simulink model "Trajectory_Tracking_comparison_v22b"  (R2022b)
settings: Solver=VariableStepAuto  StartTime=0.0  StopTime=100  RelTol=1e-3
undefined symbols (not defined in the file): A, A_uns, B, B_uns, den_phi, den_theta, K_lq_track, K_lq_track_uns, K_lq_uns, K_pp, K_pp_uns, Kd_theta, Ki_phi, Ki_theta, Kp_phi, Kp_theta, num_phi, num_theta, Va_bar, x1_bar, x1_bar_uns, x3_bar, x3_bar_uns
libraries: simulink_extras x13, slpidlib x2, simulink x1
settings Model: Creator=Mark  LastModifiedBy=Mark
settings OptimizationCC: ReuseModelBlockBuffer=on

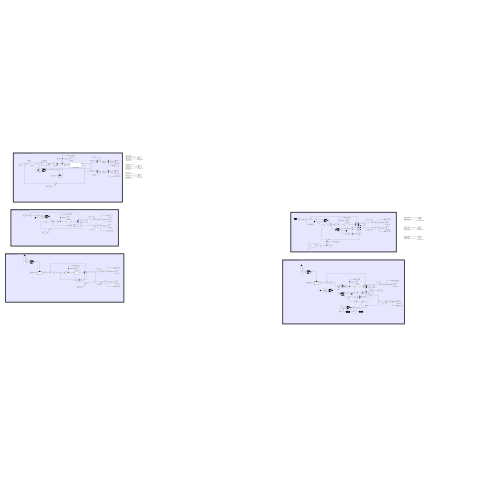
[thumbnail: Simulink's stored preview of the top-level diagram]
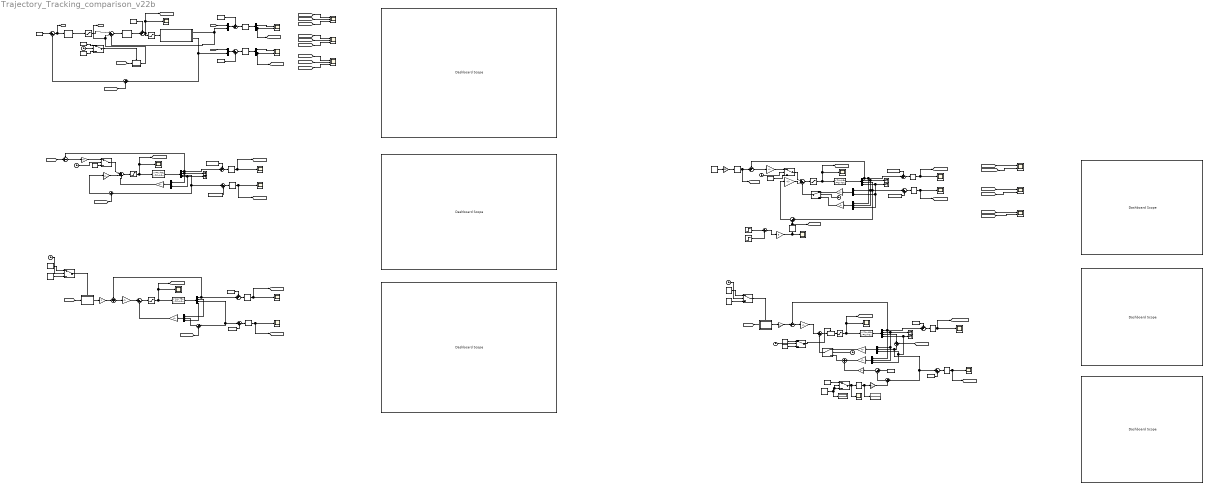
== system Trajectory_Tracking_comparison_v22b ==
  note: LQR + Trajectory Tracking at 0°
  note: LQR + Tracking Control for theta at 180°
  note: 2-DOF PID + Trajectory Tracking Control at 0°
  note: Pole Placement + Trajectory Tracking at 180°
  note: Pole Placement + Trajectory Tracking at 0°
  Clock{,1..7} (8 alike) : Clock
  Constant : Constant  Value=x3_bar_uns
  Constant1 : Constant  Value=x1_bar_uns
  Constant{2,6,10..11} (4 alike) : Constant
  Constant{3,7,12..13,19,22} (6 alike) : Constant  Value=0
  Constant14 : Constant  Value=Va_bar
  Constant15 : Constant  Value=x3_bar
  Constant16 : Constant  Value=x1_bar
  Constant17 : Constant  Value=x3_bar_uns
  Constant18 : Constant  Value=x1_bar_uns
  Constant20 : Constant  Value=x3_bar
  Constant21 : Constant  Value=x1_bar
  Constant4 : Constant  Value=pi
  Constant5 : Constant  Value=180
  Constant8 : Constant  Value=x3_bar
  Constant9 : Constant  Value=x1_bar
  Dashboard Scope{,1..5} (6 alike) : DashboardScope
  Degrees to Radians2 : simulink_extras/Transformations/Degrees to Radians
  Degrees to Radians7 : simulink_extras/Transformations/Degrees to Radians
  Degrees to Radians8 : simulink_extras/Transformations/Degrees to Radians
  Demux{,1..2,5} (4 alike) : Demux
  Demux3 : Demux  Outputs=2
  Demux4 : Demux  Outputs=2
  Display : Display
  Display1 : Display
  Enabled Subsystem : Subsystem  TreatAsAtomicUnit=on
  From : From
  Gain : Gain  Gain=[K_lq_uns(1:2) K_lq_uns(4)]  Multiplication=Matrix(K*u) (u vector)
  Gain1 : Gain  Gain=K_lq_track_uns(1)
  Gain11 : Gain  Gain=K_lq_track(1)
  Gain12 : Gain
  Gain15 : Gain  Gain=[K_pp_uns(1:2) K_pp_uns(4)]  Multiplication=Matrix(K*u) (u vector)
  Gain16 : Gain  Gain=K_pp_uns(3)
  Gain17 : Gain  Gain=K_pp(1)
  Gain18 : Gain  Gain=30
  Gain19 : Gain  Gain=K_pp_uns(1)
  Gain2 : Gain  Gain=K_lq_uns(3)
  Gain20 : Gain  Gain=[K_pp_uns(2) K_pp_uns(4)]  Multiplication=Matrix(K*u) (u vector)
  Gain21 : Gain  Gain=[K_pp(2) K_pp(4)]  Multiplication=Matrix(K*u) (u vector)
  Gain22 : Gain  Gain=5
  Gain23 : Gain  Gain=K_pp(3)
  Gain3 : Gain  Gain=K_lq_track_uns(2:4)  Multiplication=Matrix(K*u) (u vector)
  Gain4 : Gain
  Gain7 : Gain
  Gain8 : Gain  Gain=K_lq_track(2:4)  Multiplication=Matrix(K*u) (u vector)
  Mux{,1..2,6} (4 alike) : Mux  Inputs=3
  Mux{3..5,7} (4 alike) : Mux  Inputs=2
  PID_phi : slpidlib/PID Controller  Controller=I  Form=Parallel  TimeDomain=Continuous-time  UseExternalTs=off  SampleTime=-1  IntegratorMethod=Forward Euler  FilterMethod=Forward Euler  ControllerParametersSource=internal  P=Kp_phi  I=Ki_phi  UseKiTs=off  D=1  N=100  UseFilter=on  TunerSelectOption=Transfer Function Based (PID Tuner App)  InitialConditionSource=internal  InitialConditionForIntegrator=0  InitialConditionForFilter=0  DifferentiatorICPrevScaledInput=0  ExternalReset=none  TrackingMode=off  Kt=1  LimitOutput=off  SatLimitsSource=internal  UpperSaturationLimit=90  LowerSaturationLimit=-90  LinearizeAsGain=on  AntiWindupMode=none  Kb=1  LimitIntegrator=off  UpperIntegratorSaturationLimit=inf  LowerIntegratorSaturationLimit=-inf  POutMin=[]  POutMax=[]  IOutMin=[]  IOutMax=[]  DOutMin=[]  DOutMax=[]  NOutMin=[]  NOutMax=[]  SumOutMin=[]  SumOutMax=[]  SaturationOutMin=[]  SaturationOutMax=[]  PParamMin=[]  PParamMax=[]  IParamMin=[]  IParamMax=[]  DParamMin=[]  DParamMax=[]  NParamMin=[]  NParamMax=[]  KbParamMin=[]  KbParamMax=[]  KtParamMin=[]  KtParamMax=[]  KbOutMin=[]  KbOutMax=[]  KtOutMin=[]  KtOutMax=[]  IntegratorOutMin=[]  IntegratorOutMax=[]  FilterOutMin=[]  FilterOutMax=[]  SumI1OutMin=[]  SumI1OutMax=[]  SumI2OutMin=[]  SumI2OutMax=[]  SumI3OutMin=[]  SumI3OutMax=[]  SumI4OutMin=[]  SumI4OutMax=[]  SumDOutMin=[]  SumDOutMax=[]  DifferentiatorOutMin=[]  DifferentiatorOutMax=[]  FilterDiffOutCoefMin=[]  FilterDiffOutCoefMax=[]  ReciprocalOutMin=[]  ReciprocalOutMax=[]  SumDenOutMin=[]  SumDenOutMax=[]  SumNumOutMin=[]  SumNumOutMax=[]  DivideOutMin=[]  DivideOutMax=[]  UdiffTsProdOutMin=[]  UdiffTsProdOutMax=[]  NTsProdOutMin=[]  NTsProdOutMax=[]  UintegralTsProdOutMin=[]  UintegralTsProdOutMax=[]  UngainTsProdOutMin=[]  UngainTsProdOutMax=[]  IntegratorContinuousStateAttributes=''  IntegratorStateMustResolveToSignalObject=off  IntegratorRTWStateStorageClass=Auto  FilterContinuousStateAttributes=''  FilterStateMustResolveToSignalObject=off  FilterRTWStateStorageClass=Auto  ParallelPVariant=Disabled  IdealPVariant=Disabled  IVariant=InternalParameters  DVariant=Disabled  IntegratorVariant=Continuous  SatVariant=Disabled  AWVariant=Passthrough  PCopyVariant=Disabled  TRVariant=Disabled  FdbkBlocksVariant=Forward  IdealPFdbkVariant=Disabled  SatFdbkVariant=Disabled  DerivativeFilterVariant=Disabled  NVariant=Disabled  NCopyVariant=Disabled_SignalSpec  FilterICVariant=Disabled  IntegratorICVariant=InternalICs  ExternalResetVariant=Disabled  TRSumVariant=Passthrough  SumFdbkVariant=Disabled  SumVariant=Passthrough_I  TsampFilterVariant=InternalTs  TsampNgainVariant=Passthrough  TsampIntegralVariant=Disabled_SignalSpec  ExternalSaturationOutDataTypeStr=Inherit: Same as second input
  PID_theta : slpidlib/PID Controller  Controller=PID  Form=Parallel  TimeDomain=Continuous-time  UseExternalTs=off  SampleTime=-1  IntegratorMethod=Forward Euler  FilterMethod=Forward Euler  ControllerParametersSource=internal  P=Kp_theta  I=Ki_theta  UseKiTs=off  D=Kd_theta  N=100  UseFilter=on  TunerSelectOption=Transfer Function Based (PID Tuner App)  InitialConditionSource=internal  InitialConditionForIntegrator=0  InitialConditionForFilter=0  DifferentiatorICPrevScaledInput=0  ExternalReset=none  TrackingMode=off  Kt=1  LimitOutput=on  SatLimitsSource=internal  UpperSaturationLimit=10  LowerSaturationLimit=-10  LinearizeAsGain=on  AntiWindupMode=back-calculation  Kb=Ki_theta/Kp_theta  LimitIntegrator=off  UpperIntegratorSaturationLimit=inf  LowerIntegratorSaturationLimit=-inf  POutMin=[]  POutMax=[]  IOutMin=[]  IOutMax=[]  DOutMin=[]  DOutMax=[]  NOutMin=[]  NOutMax=[]  SumOutMin=[]  SumOutMax=[]  SaturationOutMin=[]  SaturationOutMax=[]  PParamMin=[]  PParamMax=[]  IParamMin=[]  IParamMax=[]  DParamMin=[]  DParamMax=[]  NParamMin=[]  NParamMax=[]  KbParamMin=[]  KbParamMax=[]  KtParamMin=[]  KtParamMax=[]  KbOutMin=[]  KbOutMax=[]  KtOutMin=[]  KtOutMax=[]  IntegratorOutMin=[]  IntegratorOutMax=[]  FilterOutMin=[]  FilterOutMax=[]  SumI1OutMin=[]  SumI1OutMax=[]  SumI2OutMin=[]  SumI2OutMax=[]  SumI3OutMin=[]  SumI3OutMax=[]  SumI4OutMin=[]  SumI4OutMax=[]  SumDOutMin=[]  SumDOutMax=[]  DifferentiatorOutMin=[]  DifferentiatorOutMax=[]  FilterDiffOutCoefMin=[]  FilterDiffOutCoefMax=[]  ReciprocalOutMin=[]  ReciprocalOutMax=[]  SumDenOutMin=[]  SumDenOutMax=[]  SumNumOutMin=[]  SumNumOutMax=[]  DivideOutMin=[]  DivideOutMax=[]  UdiffTsProdOutMin=[]  UdiffTsProdOutMax=[]  NTsProdOutMin=[]  NTsProdOutMax=[]  UintegralTsProdOutMin=[]  UintegralTsProdOutMax=[]  UngainTsProdOutMin=[]  UngainTsProdOutMax=[]  IntegratorContinuousStateAttributes=''  IntegratorStateMustResolveToSignalObject=off  IntegratorRTWStateStorageClass=Auto  FilterContinuousStateAttributes=''  FilterStateMustResolveToSignalObject=off  FilterRTWStateStorageClass=Auto  ParallelPVariant=InternalParameters  IdealPVariant=Disabled  IVariant=InternalParameters  DVariant=InternalParameters  IntegratorVariant=Continuous  SatVariant=Enabled  AWVariant=BackCalculation  PCopyVariant=Disabled  TRVariant=Disabled  FdbkBlocksVariant=Forward  IdealPFdbkVariant=Disabled  SatFdbkVariant=Disabled  DerivativeFilterVariant=ContFilter  NVariant=InternalParameters  NCopyVariant=Disabled  FilterICVariant=InternalICsFilter  IntegratorICVariant=InternalICs  ExternalResetVariant=Disabled  TRSumVariant=Passthrough  SumFdbkVariant=Disabled  SumVariant=Sum_PID  TsampFilterVariant=InternalTs  TsampNgainVariant=Passthrough  TsampIntegralVariant=Disabled_SignalSpec  ExternalSaturationOutDataTypeStr=Inherit: Same as second input
  Radians to Degrees{,1..7} (8 alike) : simulink_extras/Transformations/Radians to Degrees
  Rotary Pendulum : Subsystem
  Saturation : Saturate  UpperLimit=pi/2  LowerLimit=-pi/2
  Saturation{1..5} (5 alike) : Saturate  UpperLimit=10  LowerLimit=-10
  Scope : Scope
  Scope6 : Scope
  Signal Generator1 : SignalGenerator  Frequency=0.05
  State-Space1 : StateSpace  A=A  B=B  C=eye(4)  D=zeros(4,1)  InitialCondition=[0 0 0 0]
  State-Space2 : StateSpace  A=A_uns  B=B_uns  C=eye(4)  D=zeros(4,1)  InitialCondition=[0 0 0 0]
  State-Space3 : StateSpace  A=A  B=B  C=eye(4)  D=zeros(4,1)  InitialCondition=[0 0 0 0]
  State-Space4 : StateSpace  A=A_uns  B=B_uns  C=eye(4)  D=zeros(4,1)  InitialCondition=[0 0 0 0]  ParameterTunability=Optimized
  Step8 : Step  Time=30  SampleTime=0
  Step9 : Step  Time=30.05  SampleTime=0
  Subsystem : Subsystem
  Subsystem1 : Subsystem
  Subsystem2 : Subsystem
  Sum{,5,12,16,29} (5 alike) : Sum  Inputs=|+-
  Sum{1,13,21,23,25,32} (6 alike) : Sum  Inputs=++|
  Sum11 : Sum  Inputs=|++-
  Sum{2,6,9,14..15,19..20,27..28,33..34} (11 alike) : Sum  Inputs=|++
  Sum{4,17,26,30} (4 alike) : Sum  Inputs=-+|
  Sum24 : Sum  Inputs=|+--
  Sum31 : Sum  Inputs=|+--
  Sum8 : Sum  Inputs=|-+
  Switch{,1,4..5} (4 alike) : Switch  Criteria=u2 > Threshold  Threshold=10  SaturateOnIntegerOverflow=off  InputSameDT=off
  Switch2 : Switch  Threshold=180  SaturateOnIntegerOverflow=off  InputSameDT=off
  Switch3 : Switch  Criteria=u2 > Threshold  Threshold=5  SaturateOnIntegerOverflow=off  InputSameDT=off
  Switch6 : Switch  Threshold=10  SaturateOnIntegerOverflow=off  InputSameDT=off
  Switch7 : Switch  Threshold=10  SaturateOnIntegerOverflow=off  InputSameDT=off
  Switch8 : Switch  Threshold=10  SaturateOnIntegerOverflow=off  InputSameDT=off
  Terminator{,1..5} (6 alike) : Terminator
  Va_180 : Scope
  Va_LQR_0° : Scope
  Va_PID_0° : Scope
  Va_PP_0° : Scope
  Va_PP_180° : Scope
  Va_comparison : Scope  NumInputPorts=3
  Va_comparison_180° : Scope  NumInputPorts=2
  phi_LQR_0° : Scope
  phi_LQR_180° : Scope
  phi_PP_0° : Scope
  phi_PP_180° : Scope
  phi_comparison : Scope  NumInputPorts=3
  phi_comparison_180° : Scope  NumInputPorts=2
  phi_deg : simulink_extras/Transformations/Radians to Degrees
  phi_ramp : simulink/Sources/Ramp  slope=50  start=0  InitialOutput=0
  phi_ref1 : Constant  Value=0
  phi_sim_PID : Scope  NumInputPorts=2
  theta_LQR_0° : Scope
  theta_LQR_180° : Scope
  theta_PP_0° : Scope
  theta_PP_180° : Scope
  theta_comparison : Scope  NumInputPorts=3
  theta_comparison_180° : Scope  NumInputPorts=2
  theta_deg : simulink_extras/Transformations/Radians to Degrees
  theta_ref : Goto
  theta_sim_PID : Scope  NumInputPorts=2
  wires:
  Gain1/1 -> Sum/1
  Sum9/1 -> Mux/2, Sum2/1, Sum6/1
  Constant12/1 -> Switch4/3
  Gain11/1 -> Sum16/1
  Clock3/1 -> Switch4/2
  Saturation2/1 -> State-Space1/1, [Va_LQR_0], Va_LQR_0°/1  "Va_LQR_0°"
  Radians to Degrees2/1 -> [theta_LQR_0], theta_LQR_0°/1  "theta_LQR_0°"
  Constant11/1 -> Switch4/1
  Subsystem1/1(Out1) -> Gain12/1
  Gain2/1 -> Sum8/2
  Switch/1 -> Subsystem/Enable
  Degrees to Radians2/1 -> Gain7/1, Display1/1
  Gain12/1 -> Sum17/2
  Demux1/2 -> Mux2/1
  Mux1/1 -> Gain/1
  Constant3/1 -> Switch/3
  [theta_ref] -> Subsystem1/1(Input)
  Sum16/1 -> Saturation2/1
  Demux1/3 -> Sum14/1, Sum15/1
  Constant4/1 -> Sum5/1
  Sum14/1 -> Mux2/2
  Gain8/1 -> Sum16/2
  Sum17/1 -> Gain11/1
  Sum13/1 -> Radians to Degrees2/1
  Sum15/1 -> Radians to Degrees3/1
  Demux1/1 -> Sum13/2, Sum17/1
  Gain3/1 -> Switch1/1
  Constant8/1 -> Sum15/2
  Radians to Degrees3/1 -> [phi_LQR_0], phi_LQR_0°/1  "phi_LQR_0°"
  Sum6/1 -> Sum5/2
  Constant7/1 -> Switch3/3
  State-Space1/1 -> Demux1/1
  Sum5/1 -> Gain2/1
  Clock2/1 -> Switch3/2
  Constant6/1 -> Switch3/1
  phi_ramp/1 -> Display/1, Switch2/2, Switch2/3
  Radians to Degrees/1 -> [theta_LQR_180], theta_LQR_180°/1  "theta_LQR_180°"
  Gain/1 -> Sum8/1
  Switch2/1 -> Scope/1, Degrees to Radians2/1
  Constant2/1 -> Switch/1
  Clock/1 -> Switch/2
  Clock1/1 -> Switch1/2
  Demux/2 -> Terminator/1, Mux1/2, Mux/1
  Switch3/1 -> Enabled Subsystem/Enable
  Constant9/1 -> Sum13/1
  Demux1/4 -> Mux2/3
  Constant5/1 -> Switch2/1
  [theta_ref] -> Subsystem/1(Input)
  Sum4/1 -> Gain1/1
  Demux/3 -> Sum9/1
  Gain4/1 -> Sum4/2
  Sum1/1 -> Radians to Degrees/1
  Demux/4 -> Mux1/3, Mux/3, Terminator1/1
  Subsystem/1(Out1) -> Gain4/1
  Gain7/1 -> Sum6/2
  State-Space2/1 -> Demux/1
  Saturation1/1 -> State-Space2/1, [Va_LQR_180], Va_180/1  "Va_LQR_180°"
  Sum8/1 -> Switch1/3
  Sum2/1 -> Radians to Degrees1/1
  Switch4/1 -> Subsystem1/Enable
  Constant1/1 -> Sum1/1
  Enabled Subsystem/1(Out1) -> Saturation1/1
  Sum/1 -> Enabled Subsystem/1(In1)
  Demux/1 -> Mux1/1, Sum1/2, Sum4/1
  Switch1/1 -> Sum/2
  Mux/1 -> Gain3/1
  Mux2/1 -> Gain8/1
  [dist_on_phi] -> Sum9/2
  Radians to Degrees1/1 -> [phi_LQR_180], phi_LQR_180°/1  "phi_LQR_180°"
  Constant/1 -> Sum2/2
  From/1 -> Mux4/1
  Clock4/1 -> Switch5/2
  phi_deg/1 -> Demux3/1
  Saturation/1 -> Sum11/1
  Mux4/1 -> Sum23/2
  Demux4/2 -> [theta_PID_0], theta_sim_PID/2  "theta_PID_0°"
  Constant13/1 -> Switch5/3
  Switch5/1 -> Subsystem2/Enable
  theta_deg/1 -> Demux4/1
  Constant15/1 -> Sum19/2
  Subsystem2/1(Out1) -> theta_ref/1, Sum11/2
  Demux3/1 -> phi_sim_PID/1
  Rotary Pendulum/2(phi) -> Sum20/1, Mux3/2
  Demux3/2 -> [phi_PID_0], phi_sim_PID/2  "phi_PID_0°"
  Constant10/1 -> Switch5/1
  Demux4/1 -> theta_sim_PID/1
  Sum23/1 -> theta_deg/1
  Saturation3/1 -> Rotary Pendulum/1(Va)
  [B] -> Mux3/1
  Constant14/1 -> Sum21/1
  PID_theta/1 -> Sum21/2
  Sum12/1 -> PID_phi/1, [B]
  Sum11/1 -> PID_theta/1
  Sum19/1 -> phi_deg/1
  Constant16/1 -> Sum23/1
  Mux3/1 -> Sum19/1
  Rotary Pendulum/1(theta) -> Sum11/3, Mux4/2
  Sum21/1 -> Saturation3/1, [Va_PID_0], Va_PID_0°/1  "Va_PID_0°"
  PID_phi/1 -> Saturation/1
  [theta_ref] -> Subsystem2/1(In1)
  phi_ref1/1 -> Sum12/1
  Sum20/1 -> Sum12/2
  Constant22/1 -> Switch8/3
  Sum26/1 -> Gain17/1
  Mux7/1 -> Gain21/1
  Constant20/1 -> Sum34/2
  Demux5/1 -> Sum26/1, Sum32/2
  Sum34/1 -> Radians to Degrees7/1
  State-Space3/1 -> Demux5/1
  Constant21/1 -> Sum32/1
  Sum32/1 -> Radians to Degrees6/1
  Demux5/4 -> Mux7/2, Terminator5/1
  Saturation5/1 -> State-Space3/1, [Va_PP_0], Va_PP_0°/1  "Va_PP_0°"
  Radians to Degrees6/1 -> [theta_PP_0], theta_PP_0°/1  "theta_PP_0°"
  Demux5/3 -> Sum34/1, Sum33/1
  Demux5/2 -> Mux7/1, Terminator4/1
  Sum33/1 -> Gain23/1
  Sum31/1 -> Saturation5/1
  Sum29/1 -> Gain22/1
  Gain19/1 -> Switch6/1
  Demux2/3 -> Sum27/1, Sum28/1
  Sum24/1 -> Saturation4/1
  Degrees to Radians8/1 -> [theta_ref], Sum30/2
  Demux2/4 -> Terminator3/1, Mux5/2, Mux6/3
  Clock6/1 -> Switch7/2
  Gain20/1 -> Switch7/1
  Signal Generator1/1 -> Gain18/1
  Clock7/1 -> Switch8/2
  Saturation4/1 -> State-Space4/1, [Va_PP_180], Va_PP_180°/1  "Va_PP_180°"
  Radians to Degrees7/1 -> [phi_PP_0], phi_PP_0°/1  "phi_PP_0°"
  Constant18/1 -> Sum25/1
  Clock5/1 -> Switch6/2
  Demux2/1 -> Sum30/1, Mux6/1, Sum25/2
  Switch7/1 -> Sum24/3
  Sum30/1 -> Gain19/1
  Radians to Degrees4/1 -> [theta_PP_180], theta_PP_180°/1  "theta_PP_180°"
  State-Space4/1 -> Demux2/1
  Gain18/1 -> Degrees to Radians8/1
  Sum25/1 -> Radians to Degrees4/1
  [theta_ref] -> Sum26/2
  Switch6/1 -> Sum24/1
  Gain17/1 -> Switch8/1
  Radians to Degrees5/1 -> [phi_PP_180], phi_PP_180°/1  "phi_PP_180°"
  Sum27/1 -> Gain16/1
  Demux2/2 -> Mux5/1, Mux6/2, Terminator2/1
  Constant17/1 -> Sum28/2
  Gain16/1 -> Sum24/2
  Constant19/1 -> Switch6/3
  Mux6/1 -> Gain15/1
  Step9/1 -> Sum29/2
  Step8/1 -> Sum29/1
  Degrees to Radians7/1 -> [dist_on_phi], Sum27/2
  Gain22/1 -> Scope6/1, Degrees to Radians7/1
  Mux5/1 -> Gain20/1
  Gain21/1 -> Sum31/3
  Sum28/1 -> Radians to Degrees5/1
  Gain23/1 -> Sum31/2
  Gain15/1 -> Switch7/3
  Switch8/1 -> Sum31/1
  [Va_PID_0] -> Va_comparison/1
  [Va_PP_0] -> Va_comparison/2
  [Va_LQR_0] -> Va_comparison/3
  [phi_PID_0] -> phi_comparison/1
  [phi_PP_0] -> phi_comparison/2
  [phi_LQR_0] -> phi_comparison/3
  [theta_PID_0] -> theta_comparison/1
  [theta_PP_0] -> theta_comparison/2
  [theta_LQR_0] -> theta_comparison/3
  [theta_PP_180] -> theta_comparison_180°/1
  [theta_LQR_180] -> theta_comparison_180°/2
  [phi_PP_180] -> phi_comparison_180°/1
  [phi_LQR_180] -> phi_comparison_180°/2
  [Va_PP_180] -> Va_comparison_180°/1
  [Va_LQR_180] -> Va_comparison_180°/2
  [dist_on_phi] -> Sum20/2
  [dist_on_phi] -> Sum33/2
  [dist_on_phi] -> Sum14/2

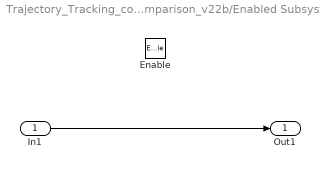
== system Trajectory_Tracking_comparison_v22b/Enabled Subsystem ==
  In1 : Inport
  Enable : EnablePort
  Out1 : Outport
  wires:
  In1/1 -> Out1/1

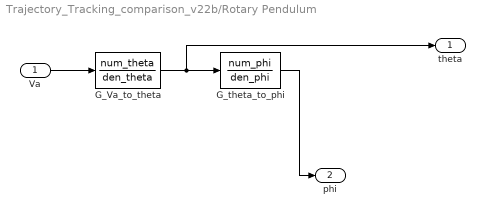
== system Trajectory_Tracking_comparison_v22b/Rotary Pendulum ==
  Va : Inport
  G_Va_to_theta : TransferFcn  Numerator=num_theta  Denominator=den_theta
  G_theta_to_phi : TransferFcn  Numerator=num_phi  Denominator=den_phi
  theta : Outport
  phi : Outport  Port=2
  wires:
  G_theta_to_phi/1 -> phi/1
  G_Va_to_theta/1 -> theta/1, G_theta_to_phi/1
  Va/1 -> G_Va_to_theta/1

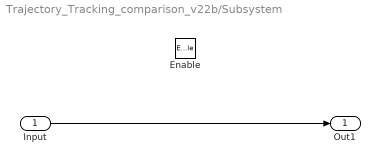
== system Trajectory_Tracking_comparison_v22b/Subsystem ==
  Input : Inport
  Enable : EnablePort
  Out1 : Outport
  wires:
  Input/1 -> Out1/1

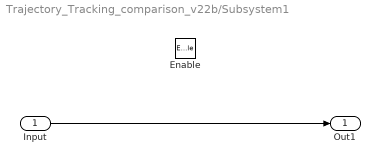
== system Trajectory_Tracking_comparison_v22b/Subsystem1 ==
  Input : Inport
  Enable : EnablePort
  Out1 : Outport
  wires:
  Input/1 -> Out1/1

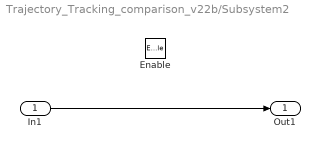
== system Trajectory_Tracking_comparison_v22b/Subsystem2 ==
  In1 : Inport
  Enable : EnablePort
  Out1 : Outport
  wires:
  In1/1 -> Out1/1
